simulink model "StateSpaceFeedback"  (R2020b)
settings: Solver=VariableStepAuto  StartTime=0.0  StopTime=10.0  RelTol=1e-3
undefined symbols (not defined in the file): A_num, B_num, C, K_with_I
settings Model: Creator=kpass  LastModifiedBy=kpass

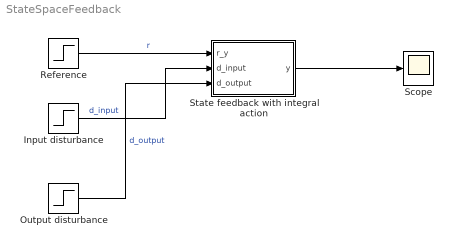
== system StateSpaceFeedback ==
  Input disturbance : Step  Time=30  SampleTime=0
  Output disturbance : Step  Time=60  SampleTime=0
  Reference : Step  SampleTime=0
  Scope : Scope
  State feedback with integral action : Subsystem
  wires:
  State feedback with integral action/1(y) -> Scope/1
  Output disturbance/1 -> State feedback with integral action/3(d_output)  "d_output"
  Reference/1 -> State feedback with integral action/1(r_y)  "r"
  Input disturbance/1 -> State feedback with integral action/2(d_input)  "d_input"

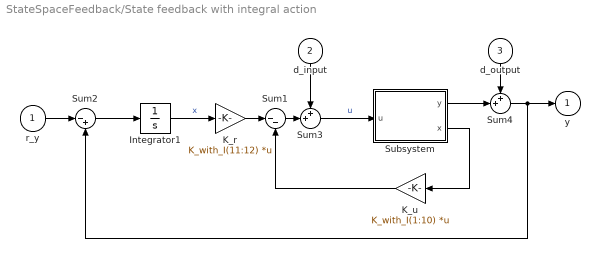
== system StateSpaceFeedback/State feedback with integral action ==
  r_y : Inport
  d_input : Inport  Port=2
  d_output : Inport  Port=3
  Integrator1 : Integrator
  K_r : Gain  Gain=K_with_I(11:12)  Multiplication=Matrix(K*u)
  K_u : Gain  Gain=K_with_I(1:10)  Multiplication=Matrix(K*u)
  Subsystem : Subsystem
  Sum1 : Sum  Inputs=|--
  Sum2 : Sum  Inputs=|-+
  Sum3 : Sum  Inputs=++|
  Sum4 : Sum  Inputs=++|
  y : Outport
  wires:
  K_u/1 -> Sum1/2
  Sum4/1 -> y/1, Sum2/2
  K_r/1 -> Sum1/1
  Sum2/1 -> Integrator1/1
  Sum1/1 -> Sum3/2
  Integrator1/1 -> K_r/1  "x"
  r_y/1 -> Sum2/1
  d_input/1 -> Sum3/1
  d_output/1 -> Sum4/1
  Sum3/1 -> Subsystem/1(u)  "u"
  Subsystem/1(y) -> Sum4/2
  Subsystem/2(x) -> K_u/1

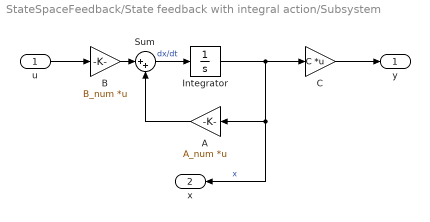
== system StateSpaceFeedback/State feedback with integral action/Subsystem ==
  u : Inport
  A : Gain  Gain=A_num  Multiplication=Matrix(K*u)
  B : Gain  Gain=B_num  Multiplication=Matrix(K*u)
  C : Gain  Gain=C  Multiplication=Matrix(K*u)
  Integrator : Integrator
  Sum : Sum  Inputs=|++
  y : Outport
  x : Outport  Port=2
  wires:
  Integrator/1 -> x/1, A/1, C/1  "x"
  u/1 -> B/1
  Sum/1 -> Integrator/1  "dx/dt"
  A/1 -> Sum/2
  C/1 -> y/1
  B/1 -> Sum/1
